simulink model "Open_Closed_LoopSystems"  (R2023b)
settings: Solver=VariableStepAuto  StartTime=0.0  StopTime=20  MaxStep=1e-3  RelTol=1e-3
libraries: simulink x4
settings Model: Creator=MOHAMED  LastModifiedBy=MOHAMED

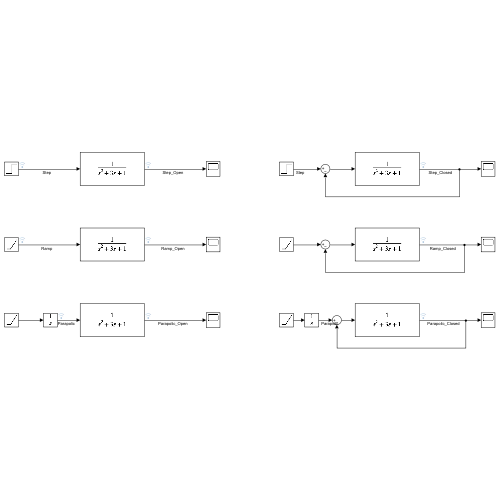
[thumbnail: Simulink's stored preview of the top-level diagram]
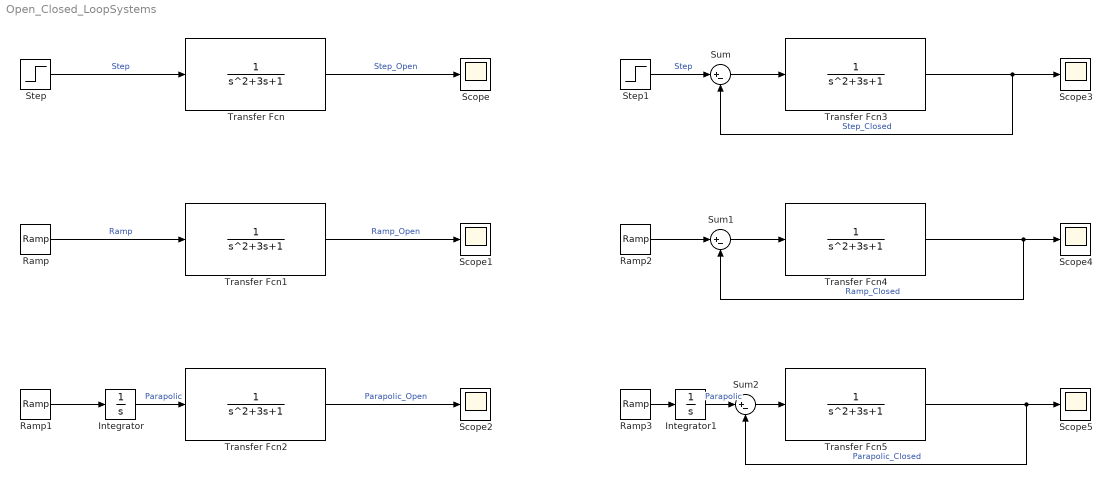
== system Open_Closed_LoopSystems ==
  Integrator : Integrator
  Integrator1 : Integrator
  Ramp{,1..3} (4 alike) : simulink/Sources/Ramp  slope=1  start=1  InitialOutput=0
  Scope{,1..5} (6 alike) : Scope
  Step : Step  SampleTime=0
  Step1 : Step  SampleTime=0
  Sum : Sum  Inputs=|+-
  Sum1 : Sum  Inputs=|+-
  Sum2 : Sum  Inputs=|+-
  Transfer Fcn{,1..5} (6 alike) : TransferFcn  Denominator=[1 3 1]
  wires:
  Step/1 -> Transfer Fcn/1  "Step"
  Transfer Fcn/1 -> Scope/1  "Step_Open"
  Transfer Fcn1/1 -> Scope1/1  "Ramp_Open"
  Ramp/1 -> Transfer Fcn1/1  "Ramp"
  Integrator/1 -> Transfer Fcn2/1  "Parapolic"
  Transfer Fcn2/1 -> Scope2/1  "Parapolic_Open"
  Ramp1/1 -> Integrator/1
  Ramp3/1 -> Integrator1/1
  Transfer Fcn5/1 -> Sum2/2, Scope5/1  "Parapolic_Closed"
  Transfer Fcn4/1 -> Sum1/2, Scope4/1  "Ramp_Closed"
  Transfer Fcn3/1 -> Sum/2, Scope3/1  "Step_Closed"
  Sum/1 -> Transfer Fcn3/1
  Step1/1 -> Sum/1  "Step"
  Sum1/1 -> Transfer Fcn4/1
  Ramp2/1 -> Sum1/1
  Integrator1/1 -> Sum2/1  "Parapolic"
  Sum2/1 -> Transfer Fcn5/1
